simulink model "sampleModel26"  (R2021b)
settings: Solver=VariableStepAuto  StartTime=0.0  StopTime=10.0  RelTol=1e-3
undefined symbols (not defined in the file or in its folder): Newton, Raphson
libraries: simulink x8, slpidlib x4
settings Model: Creator=user  LastModifiedBy=user

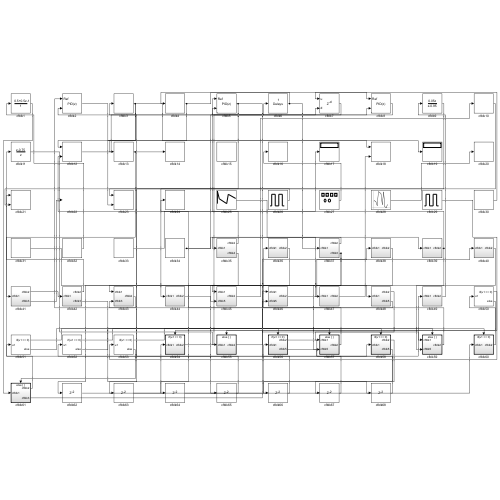
[thumbnail: Simulink's stored preview of the top-level diagram]
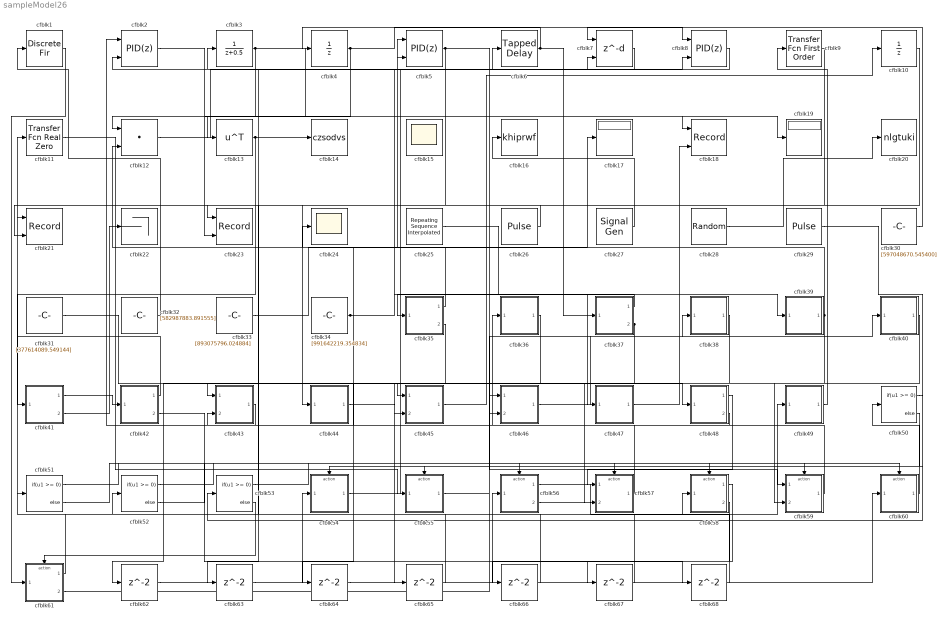
== system sampleModel26 ==
  cfblk1 : DiscreteFir  SampleTime=1
  cfblk10 : UnitDelay  HasFrameUpgradeWarning=on
  cfblk11 : simulink/Discrete/Transfer Fcn Real Zero  ZeroZ=0.75  ICPrevInput=0.0  DoSatur=off
      settings: SourceProductBaseCode=SL
  cfblk12 : DotProduct  InputSameDT=on  OutDataTypeStr=Inherit: Inherit via internal rule
  cfblk13 : Math  Operator=transpose  SaturateOnIntegerOverflow=on
  cfblk14 : ToWorkspace  VariableName=czsodvs  SaveFormat=Timeseries  SampleTime=-1
  cfblk15 : Scope
      settings: Floating=on
  cfblk16 : ToWorkspace  VariableName=khiprwf  SaveFormat=Timeseries  SampleTime=-1
  cfblk17 : Display
  cfblk18 : Record  FileSettingsInternal="{\"entries\":[{\"content\":{\"excelSettings\":{\"content\":{},\"type\":\"Streamout.ExcelSettings\"}},\"type\":\"Streamout.FileSettingStorage\",\"uuid\":\"d4ca884b-6ed6-4891-9e51-d09ac0b6b69e\"}],\"packageUris\":[\"http://schema.mathworks.com/mf0/streamout_blocks/R2020a\"],\"version\":\"1.0\"}"  Layout=[1 1]  SignalsInternal="{\"entries\":[{\"content\":{\"signals\":[{\"content\":{\"blockPath\":[\"sampleModel26/cfblk18\"],\"channel\":[],\"dimensions\":[1,1],\"domain\":\"sampleModel26/cfblk18\",\"lineColor\":\"#a2142f\",\"plots\":[1],\"port\":1,\"sid\":[\"\"],\"signalID\":1005,\"signalName\":\"cfblk3\"},\"type\":\"RecordBlkView.Signal\",\"uuid\":\"a261fcf9-e0b9-45cc-8216-5c8b8619bc2a\"},{\"content\":{\"blockPath\":[\"sampleModel26/cfblk18\"],\"channel\":[],\"dimensions\":[1],\"domain\":\"sampleModel26/cfblk18\",\"lineColor\":\"#139fff\",\"plots\":[1],\"port\":2,\"sid\":[\"\"],\"signalID\":1009,\"signalName\":\"cfblk47\"},\"type\":\"RecordBlkView.Signal\",\"uuid\":\"1b304590-a019-4fec-9271-47d6089c9687\"}]},\"type\":\"RecordBlkView.InputSignals\",\"uuid\":\"9f67ef88-f35c-4418-a645-35f536b90e1d\"}],\"packageUris\":[\"http://schema.mathworks.com/mf0/streamout_blocks/R2020a\"],\"version\":\"1.0\"}"  VisualizationBindings="{\"xyplotplugin\":{\"info\":[{\"series\":[{\"bindingParametersList\":[{\"parameter\":\"X-Axis\",\"signalID\":1005,\"signalName\":\"cfblk3\"},{\"parameter\":\"Y-Axis\",\"signalID\":1009,\"signalName\":\"cfblk47\"}],\"seriesID\":9986}],\"subplotID\":1}]}}"  CompatibilityTag=XY
  cfblk19 : Display
  cfblk2 : slpidlib/PID Controller (2DOF)  Controller=PID  Form=Parallel  TimeDomain=Discrete-time  UseExternalTs=off  SampleTime=1  IntegratorMethod=Forward Euler  FilterMethod=Forward Euler  ControllerParametersSource=internal  P=1  I=1  D=0  UseFilter=on  N=100  b=1  c=1  TunerSelectOption=Transfer Function Based (PID Tuner App)  InitialConditionSource=internal  InitialConditionForIntegrator=0  InitialConditionForFilter=0  DifferentiatorICPrevScaledInput=0  ExternalReset=none  TrackingMode=off  Kt=1  LimitOutput=off  SatLimitsSource=internal  UpperSaturationLimit=inf  LowerSaturationLimit=-inf  LinearizeAsGain=off  AntiWindupMode=none  Kb=1  POutMin=[]  POutMax=[]  IOutMin=[]  IOutMax=[]  DOutMin=[]  DOutMax=[]  NOutMin=[]  NOutMax=[]  bOutMin=[]  bOutMax=[]  cOutMin=[]  cOutMax=[]  SumOutMin=[]  SumOutMax=[]  SaturationOutMin=[]  SaturationOutMax=[]  PParamMin=[]  PParamMax=[]  IParamMin=[]  IParamMax=[]  DParamMin=[]  DParamMax=[]  NParamMin=[]  NParamMax=[]  bParamMin=[]  bParamMax=[]  cParamMin=[]  cParamMax=[]  KbParamMin=[]  KbParamMax=[]  KtParamMin=[]  KtParamMax=[]  KbOutMin=[]  KbOutMax=[]  KtOutMin=[]  KtOutMax=[]  IntegratorOutMin=[]  IntegratorOutMax=[]  FilterOutMin=[]  FilterOutMax=[]  SumI1OutMin=[]  SumI1OutMax=[]  SumI2OutMin=[]  SumI2OutMax=[]  SumI3OutMin=[]  SumI3OutMax=[]  SumI4OutMin=[]  SumI4OutMax=[]  SumDOutMin=[]  SumDOutMax=[]  Sum1OutMin=[]  Sum1OutMax=[]  Sum2OutMin=[]  Sum2OutMax=[]  Sum3OutMin=[]  Sum3OutMax=[]  DifferentiatorOutMin=[]  DifferentiatorOutMax=[]  FilterDiffOutCoefMin=[]  FilterDiffOutCoefMax=[]  ReciprocalOutMin=[]  ReciprocalOutMax=[]  SumDenOutMin=[]  SumDenOutMax=[]  SumNumOutMin=[]  SumNumOutMax=[]  DivideOutMin=[]  DivideOutMax=[]  UdiffTsProdOutMin=[]  UdiffTsProdOutMax=[]  NTsProdOutMin=[]  NTsProdOutMax=[]  UintegralTsProdOutMin=[]  UintegralTsProdOutMax=[]  UngainTsProdOutMin=[]  UngainTsProdOutMax=[]  IntegratorContinuousStateAttributes=''  IntegratorStateMustResolveToSignalObject=off  IntegratorRTWStateStorageClass=Auto  FilterContinuousStateAttributes=''  FilterStateMustResolveToSignalObject=off  FilterRTWStateStorageClass=Auto  ParallelPVariant=InternalParameters  IdealPVariant=Disabled  IVariant=InternalParameters  DVariant=InternalParameters  bVariant=InternalParameters  cVariant=InternalParameters  IntegratorVariant=Discrete  SatVariant=Disabled  AWVariant=Passthrough  PCopyVariant=Disabled  TRVariant=Disabled  FdbkBlocksVariant=Forward  IdealPFdbkVariant=Disabled  SatFdbkVariant=Disabled  DerivativeFilterVariant=ForwardEulerFilter  NVariant=InternalParameters  NCopyVariant=Disabled  FilterICVariant=InternalICsFilter  IntegratorICVariant=InternalICs  ExternalResetVariant=Disabled  TRSumVariant=Passthrough  SumFdbkVariant=Disabled  SumVariant=Sum_PID  TsampFilterVariant=InternalTs  TsampNgainVariant=Passthrough  TsampIntegralVariant=Passthrough  ExternalSaturationOutDataTypeStr=Inherit: Same as second input
      settings: SourceProductBaseCode=SL
  cfblk20 : ToWorkspace  VariableName=nlgtuki  SaveFormat=Timeseries  SampleTime=-1
  cfblk21 : Record  FileSettingsInternal="{\"entries\":[{\"content\":{\"excelSettings\":{\"content\":{},\"type\":\"Streamout.ExcelSettings\"}},\"type\":\"Streamout.FileSettingStorage\",\"uuid\":\"902d94bf-6ad9-4d8d-bb43-3e97950e27a8\"}],\"packageUris\":[\"http://schema.mathworks.com/mf0/streamout_blocks/R2020a\"],\"version\":\"1.0\"}"  Layout=[1 1]  SignalsInternal="{\"entries\":[{\"content\":{\"signals\":[{\"content\":{\"blockPath\":[\"sampleModel26/cfblk21\"],\"channel\":[],\"dimensions\":[1,1],\"domain\":\"sampleModel26/cfblk21\",\"lineColor\":\"#a2142f\",\"plots\":[1],\"port\":1,\"sid\":[\"\"],\"signalID\":1013,\"signalName\":\"cfblk42:1\"},\"type\":\"RecordBlkView.Signal\",\"uuid\":\"12224121-8beb-4598-b1fb-51b9937be4c3\"},{\"content\":{\"blockPath\":[\"sampleModel26/cfblk21\"],\"channel\":[],\"dimensions\":[1],\"domain\":\"sampleModel26/cfblk21\",\"lineColor\":\"#139fff\",\"plots\":[1],\"port\":2,\"sid\":[\"\"],\"signalID\":1017,\"signalName\":\"cfblk10\"},\"type\":\"RecordBlkView.Signal\",\"uuid\":\"13295fa7-14f4-4ec2-bdc1-d2cd68b79197\"}]},\"type\":\"RecordBlkView.InputSignals\",\"uuid\":\"09763a43-9cb4-444a-8828-0097ae43f352\"}],\"packageUris\":[\"http://schema.mathworks.com/mf0/streamout_blocks/R2020a\"],\"version\":\"1.0\"}"  VisualizationBindings="{\"xyplotplugin\":{\"info\":[{\"series\":[{\"bindingParametersList\":[{\"parameter\":\"X-Axis\",\"signalID\":1013,\"signalName\":\"cfblk42:1\"},{\"parameter\":\"Y-Axis\",\"signalID\":1017,\"signalName\":\"cfblk10\"}],\"seriesID\":13624}],\"subplotID\":1}]}}"  CompatibilityTag=XY
  cfblk22 : Terminator
  cfblk23 : Record  FileSettingsInternal="{\"entries\":[{\"content\":{\"excelSettings\":{\"content\":{},\"type\":\"Streamout.ExcelSettings\"}},\"type\":\"Streamout.FileSettingStorage\",\"uuid\":\"a11609d8-2a1b-417e-a440-ff965ac5fa11\"}],\"packageUris\":[\"http://schema.mathworks.com/mf0/streamout_blocks/R2020a\"],\"version\":\"1.0\"}"  Layout=[1 1]  SignalsInternal="{\"entries\":[{\"content\":{\"signals\":[{\"content\":{\"blockPath\":[\"sampleModel26/cfblk23\"],\"channel\":[],\"dimensions\":[1],\"domain\":\"sampleModel26/cfblk23\",\"lineColor\":\"#a2142f\",\"plots\":[1],\"port\":1,\"sid\":[\"\"],\"signalID\":1021,\"signalName\":\"cfblk26\"},\"type\":\"RecordBlkView.Signal\",\"uuid\":\"2700e2c5-e2e7-479b-8112-f551c1b5b9e0\"},{\"content\":{\"blockPath\":[\"sampleModel26/cfblk23\"],\"channel\":[],\"dimensions\":[1,1],\"domain\":\"sampleModel26/cfblk23\",\"lineColor\":\"#139fff\",\"plots\":[1],\"port\":2,\"sid\":[\"\"],\"signalID\":1025,\"signalName\":\"cfblk3\"},\"type\":\"RecordBlkView.Signal\",\"uuid\":\"01e7d8b1-2d56-4034-97cc-cc956fd5e74b\"}]},\"type\":\"RecordBlkView.InputSignals\",\"uuid\":\"823d7022-7059-491d-bee7-1f860ba1237c\"}],\"packageUris\":[\"http://schema.mathworks.com/mf0/streamout_blocks/R2020a\"],\"version\":\"1.0\"}"  VisualizationBindings="{\"xyplotplugin\":{\"info\":[{\"series\":[{\"bindingParametersList\":[{\"parameter\":\"X-Axis\",\"signalID\":1021,\"signalName\":\"cfblk26\"},{\"parameter\":\"Y-Axis\",\"signalID\":1025,\"signalName\":\"cfblk3\"}],\"seriesID\":28488}],\"subplotID\":1}]}}"  CompatibilityTag=XY
  cfblk24 : Scope
  cfblk25 : simulink/Sources/Repeating Sequence Interpolated  OutValues=[-38149698.186429, -442988164.448479, -683927649.777651, -209183975.881470, -429087904.669824]  TimeValues=[0 0.1 0.5 0.6 1].'  LookUpMeth=Interpolation-Use End Values  tsamp=0.01  OutMin=[]  OutMax=[]  OutDataTypeStr=double  OutputDataTypeScalingMode=double  OutDataType=fixdt(0,8)  OutScaling=2^-10
  cfblk26 : DiscretePulseGenerator  PulseType=Time based  Amplitude=[285039313.385840]  Period=[95692373.632031]  PulseWidth=5  PhaseDelay=[2.000000]
  cfblk27 : SignalGenerator  WaveForm=square  Amplitude=[819033828.996605]  Units=rad/sec
  cfblk28 : RandomNumber  Mean=[40847.688215]  Variance=[65157.945720]  Seed=[331896928.000000]  SampleTime=0.1
  cfblk29 : DiscretePulseGenerator  PulseType=Time based  Amplitude=[43137341.195168]  Period=[2476344.846735]  PulseWidth=5  PhaseDelay=[1.000000]
  cfblk3 : DiscreteTransferFcn  SampleTime=1
  cfblk30 : Constant  Value=[597048670.545400]  SampleTime=1
  cfblk31 : Constant  Value=[377614089.549144]  SampleTime=1
  cfblk32 : Constant  Value=[582987883.891555]  SampleTime=1
  cfblk33 : Constant  Value=[893075796.024884]  SampleTime=1
  cfblk34 : Constant  Value=[991642219.354834]  SampleTime=1
  cfblk35 : Subsystem
  cfblk36 : Subsystem
  cfblk37 : Subsystem
  cfblk38 : Subsystem
  cfblk39 : Subsystem
  cfblk4 : UnitDelay  HasFrameUpgradeWarning=on
  cfblk40 : Subsystem
  cfblk41 : Subsystem
  cfblk42 : Subsystem
  cfblk43 : Subsystem
  cfblk44 : Subsystem
  cfblk45 : Subsystem
  cfblk46 : Subsystem
  cfblk47 : Subsystem
  cfblk48 : Subsystem
  cfblk49 : Subsystem
  cfblk5 : slpidlib/PID Controller (2DOF)  Controller=PID  Form=Parallel  TimeDomain=Discrete-time  UseExternalTs=off  SampleTime=1  IntegratorMethod=Forward Euler  FilterMethod=Forward Euler  ControllerParametersSource=internal  P=1  I=1  D=0  UseFilter=on  N=100  b=1  c=1  TunerSelectOption=Transfer Function Based (PID Tuner App)  InitialConditionSource=internal  InitialConditionForIntegrator=0  InitialConditionForFilter=0  DifferentiatorICPrevScaledInput=0  ExternalReset=none  TrackingMode=off  Kt=1  LimitOutput=off  SatLimitsSource=internal  UpperSaturationLimit=inf  LowerSaturationLimit=-inf  LinearizeAsGain=off  AntiWindupMode=none  Kb=1  POutMin=[]  POutMax=[]  IOutMin=[]  IOutMax=[]  DOutMin=[]  DOutMax=[]  NOutMin=[]  NOutMax=[]  bOutMin=[]  bOutMax=[]  cOutMin=[]  cOutMax=[]  SumOutMin=[]  SumOutMax=[]  SaturationOutMin=[]  SaturationOutMax=[]  PParamMin=[]  PParamMax=[]  IParamMin=[]  IParamMax=[]  DParamMin=[]  DParamMax=[]  NParamMin=[]  NParamMax=[]  bParamMin=[]  bParamMax=[]  cParamMin=[]  cParamMax=[]  KbParamMin=[]  KbParamMax=[]  KtParamMin=[]  KtParamMax=[]  KbOutMin=[]  KbOutMax=[]  KtOutMin=[]  KtOutMax=[]  IntegratorOutMin=[]  IntegratorOutMax=[]  FilterOutMin=[]  FilterOutMax=[]  SumI1OutMin=[]  SumI1OutMax=[]  SumI2OutMin=[]  SumI2OutMax=[]  SumI3OutMin=[]  SumI3OutMax=[]  SumI4OutMin=[]  SumI4OutMax=[]  SumDOutMin=[]  SumDOutMax=[]  Sum1OutMin=[]  Sum1OutMax=[]  Sum2OutMin=[]  Sum2OutMax=[]  Sum3OutMin=[]  Sum3OutMax=[]  DifferentiatorOutMin=[]  DifferentiatorOutMax=[]  FilterDiffOutCoefMin=[]  FilterDiffOutCoefMax=[]  ReciprocalOutMin=[]  ReciprocalOutMax=[]  SumDenOutMin=[]  SumDenOutMax=[]  SumNumOutMin=[]  SumNumOutMax=[]  DivideOutMin=[]  DivideOutMax=[]  UdiffTsProdOutMin=[]  UdiffTsProdOutMax=[]  NTsProdOutMin=[]  NTsProdOutMax=[]  UintegralTsProdOutMin=[]  UintegralTsProdOutMax=[]  UngainTsProdOutMin=[]  UngainTsProdOutMax=[]  IntegratorContinuousStateAttributes=''  IntegratorStateMustResolveToSignalObject=off  IntegratorRTWStateStorageClass=Auto  FilterContinuousStateAttributes=''  FilterStateMustResolveToSignalObject=off  FilterRTWStateStorageClass=Auto  ParallelPVariant=InternalParameters  IdealPVariant=Disabled  IVariant=InternalParameters  DVariant=InternalParameters  bVariant=InternalParameters  cVariant=InternalParameters  IntegratorVariant=Discrete  SatVariant=Disabled  AWVariant=Passthrough  PCopyVariant=Disabled  TRVariant=Disabled  FdbkBlocksVariant=Forward  IdealPFdbkVariant=Disabled  SatFdbkVariant=Disabled  DerivativeFilterVariant=ForwardEulerFilter  NVariant=InternalParameters  NCopyVariant=Disabled  FilterICVariant=InternalICsFilter  IntegratorICVariant=InternalICs  ExternalResetVariant=Disabled  TRSumVariant=Passthrough  SumFdbkVariant=Disabled  SumVariant=Sum_PID  TsampFilterVariant=InternalTs  TsampNgainVariant=Passthrough  TsampIntegralVariant=Passthrough  ExternalSaturationOutDataTypeStr=Inherit: Same as second input
      settings: SourceProductBaseCode=SL
  cfblk{50..53} (4 alike) : If  IfExpression=u1 >= 0  SampleTime=1
  cfblk54 : Subsystem  TreatAsAtomicUnit=on
  cfblk55 : Subsystem  TreatAsAtomicUnit=on
  cfblk56 : Subsystem  TreatAsAtomicUnit=on
  cfblk57 : Subsystem  TreatAsAtomicUnit=on
  cfblk58 : Subsystem  TreatAsAtomicUnit=on
  cfblk59 : Subsystem  TreatAsAtomicUnit=on
  cfblk6 : simulink/Discrete/Tapped Delay  vinit=0.0  samptime=-1  NumDelays=1  DelayOrder=Oldest  includeCurrent=off
  cfblk60 : Subsystem  TreatAsAtomicUnit=on
  cfblk61 : Subsystem  TreatAsAtomicUnit=on
  cfblk{62..68} (7 alike) : Delay  SampleTime=1
  cfblk7 : Delay  DelayLengthSource=Input port  SampleTime=1
      settings: InputPortMap=u0,p1
  cfblk8 : slpidlib/PID Controller (2DOF)  Controller=PID  Form=Parallel  TimeDomain=Discrete-time  UseExternalTs=off  SampleTime=1  IntegratorMethod=Forward Euler  FilterMethod=Forward Euler  ControllerParametersSource=internal  P=1  I=1  D=0  UseFilter=on  N=100  b=1  c=1  TunerSelectOption=Transfer Function Based (PID Tuner App)  InitialConditionSource=internal  InitialConditionForIntegrator=0  InitialConditionForFilter=0  DifferentiatorICPrevScaledInput=0  ExternalReset=none  TrackingMode=off  Kt=1  LimitOutput=off  SatLimitsSource=internal  UpperSaturationLimit=inf  LowerSaturationLimit=-inf  LinearizeAsGain=off  AntiWindupMode=none  Kb=1  POutMin=[]  POutMax=[]  IOutMin=[]  IOutMax=[]  DOutMin=[]  DOutMax=[]  NOutMin=[]  NOutMax=[]  bOutMin=[]  bOutMax=[]  cOutMin=[]  cOutMax=[]  SumOutMin=[]  SumOutMax=[]  SaturationOutMin=[]  SaturationOutMax=[]  PParamMin=[]  PParamMax=[]  IParamMin=[]  IParamMax=[]  DParamMin=[]  DParamMax=[]  NParamMin=[]  NParamMax=[]  bParamMin=[]  bParamMax=[]  cParamMin=[]  cParamMax=[]  KbParamMin=[]  KbParamMax=[]  KtParamMin=[]  KtParamMax=[]  KbOutMin=[]  KbOutMax=[]  KtOutMin=[]  KtOutMax=[]  IntegratorOutMin=[]  IntegratorOutMax=[]  FilterOutMin=[]  FilterOutMax=[]  SumI1OutMin=[]  SumI1OutMax=[]  SumI2OutMin=[]  SumI2OutMax=[]  SumI3OutMin=[]  SumI3OutMax=[]  SumI4OutMin=[]  SumI4OutMax=[]  SumDOutMin=[]  SumDOutMax=[]  Sum1OutMin=[]  Sum1OutMax=[]  Sum2OutMin=[]  Sum2OutMax=[]  Sum3OutMin=[]  Sum3OutMax=[]  DifferentiatorOutMin=[]  DifferentiatorOutMax=[]  FilterDiffOutCoefMin=[]  FilterDiffOutCoefMax=[]  ReciprocalOutMin=[]  ReciprocalOutMax=[]  SumDenOutMin=[]  SumDenOutMax=[]  SumNumOutMin=[]  SumNumOutMax=[]  DivideOutMin=[]  DivideOutMax=[]  UdiffTsProdOutMin=[]  UdiffTsProdOutMax=[]  NTsProdOutMin=[]  NTsProdOutMax=[]  UintegralTsProdOutMin=[]  UintegralTsProdOutMax=[]  UngainTsProdOutMin=[]  UngainTsProdOutMax=[]  IntegratorContinuousStateAttributes=''  IntegratorStateMustResolveToSignalObject=off  IntegratorRTWStateStorageClass=Auto  FilterContinuousStateAttributes=''  FilterStateMustResolveToSignalObject=off  FilterRTWStateStorageClass=Auto  ParallelPVariant=InternalParameters  IdealPVariant=Disabled  IVariant=InternalParameters  DVariant=InternalParameters  bVariant=InternalParameters  cVariant=InternalParameters  IntegratorVariant=Discrete  SatVariant=Disabled  AWVariant=Passthrough  PCopyVariant=Disabled  TRVariant=Disabled  FdbkBlocksVariant=Forward  IdealPFdbkVariant=Disabled  SatFdbkVariant=Disabled  DerivativeFilterVariant=ForwardEulerFilter  NVariant=InternalParameters  NCopyVariant=Disabled  FilterICVariant=InternalICsFilter  IntegratorICVariant=InternalICs  ExternalResetVariant=Disabled  TRSumVariant=Passthrough  SumFdbkVariant=Disabled  SumVariant=Sum_PID  TsampFilterVariant=InternalTs  TsampNgainVariant=Passthrough  TsampIntegralVariant=Passthrough  ExternalSaturationOutDataTypeStr=Inherit: Same as second input
      settings: SourceProductBaseCode=SL
  cfblk9 : simulink/Discrete/Transfer Fcn First Order  PoleZ=0.95  ICPrevOutput=0.0  DoSatur=off
  wires:
  cfblk46/1(cfblk2) -> cfblk38/1(cfblk1)
  cfblk57/1(cfblk2) -> cfblk36/1(cfblk1)
  cfblk54/1(cfblk2) -> cfblk6/1
  cfblk45/1(cfblk2) -> cfblk10/1
  cfblk37/1(cfblk2) -> cfblk35/1(cfblk1)
  cfblk28/1 -> cfblk20/1
  cfblk60/1(cfblk2) -> cfblk50/1
  cfblk56/1(cfblk2) -> cfblk49/1(cfblk1)
  cfblk4/1 -> cfblk12/1, cfblk8/1
  cfblk29/1 -> cfblk53/1
  cfblk13/1 -> cfblk14/1, cfblk41/1(cfblk1)
  cfblk34/1 -> cfblk39/1(cfblk1), cfblk8/2
  cfblk37/2(cfblk3) -> cfblk43/1(cfblk1), cfblk57/2(cfblk5)
  cfblk30/1 -> cfblk7/1
  cfblk3/1 -> cfblk18/1, cfblk13/1, cfblk23/2
  cfblk61/1(cfblk2) -> cfblk11/1
  cfblk48/1(cfblk2) -> cfblk57/1(cfblk1)
  cfblk39/1(cfblk2) -> cfblk5/1, cfblk59/2(cfblk5)
  cfblk43/1(cfblk2) -> cfblk2/1
  cfblk12/1 -> cfblk7/2
  cfblk31/1 -> cfblk48/1(cfblk1)
  cfblk55/1(cfblk2) -> cfblk40/1(cfblk1)
  cfblk1/1 -> cfblk61/1(cfblk1)
  cfblk33/1 -> cfblk17/1
  cfblk61/2(cfblk3) -> cfblk46/2(cfblk5)
  cfblk9/1 -> cfblk44/1(cfblk1)
  cfblk56/2(cfblk5) -> cfblk58/1(cfblk1)
  cfblk42/1(cfblk2) -> cfblk21/1
  cfblk59/1(cfblk2) -> cfblk24/1
  cfblk47/1(cfblk2) -> cfblk18/2
  cfblk11/1 -> cfblk55/1(cfblk1)
  cfblk48/2(cfblk5) -> cfblk43/2(cfblk3)
  cfblk5/1 -> cfblk59/1(cfblk1), cfblk63/1
  cfblk32/1 -> cfblk1/1
  cfblk8/1 -> cfblk2/2
  cfblk49/1(cfblk2) -> cfblk9/1
  cfblk40/1(cfblk2) -> cfblk45/1(cfblk1)
  cfblk10/1 -> cfblk21/2
  cfblk41/1(cfblk2) -> cfblk42/1(cfblk1)
  cfblk25/1 -> cfblk47/1(cfblk1)
  cfblk2/1 -> cfblk19/1
  cfblk27/1 -> cfblk16/1
  cfblk7/1 -> cfblk5/2
  cfblk35/1(cfblk2) -> cfblk12/2
  cfblk26/1 -> cfblk23/1
  cfblk6/1 -> cfblk4/1, cfblk37/1(cfblk1)
  cfblk41/2(cfblk3) -> cfblk22/1
  cfblk35/2(cfblk4) -> cfblk45/2(cfblk5)
  cfblk50/1 -> cfblk54/Action
  cfblk50/2 -> cfblk55/Action
  cfblk51/1 -> cfblk56/Action
  cfblk51/2 -> cfblk57/Action
  cfblk52/1 -> cfblk58/Action
  cfblk52/2 -> cfblk59/Action
  cfblk53/1 -> cfblk60/Action
  cfblk53/2 -> cfblk61/Action
  cfblk38/1(cfblk2) -> cfblk62/1
  cfblk62/1 -> cfblk60/1(cfblk1)
  cfblk63/1 -> cfblk54/1(cfblk1)
  cfblk36/1(cfblk2) -> cfblk64/1
  cfblk64/1 -> cfblk56/1(cfblk1)
  cfblk44/1(cfblk2) -> cfblk65/1
  cfblk65/1 -> cfblk51/1
  cfblk58/1(cfblk2) -> cfblk66/1
  cfblk66/1 -> cfblk46/1(cfblk1)
  cfblk58/2(cfblk5) -> cfblk67/1
  cfblk67/1 -> cfblk52/1
  cfblk42/2(cfblk3) -> cfblk68/1
  cfblk68/1 -> cfblk3/1

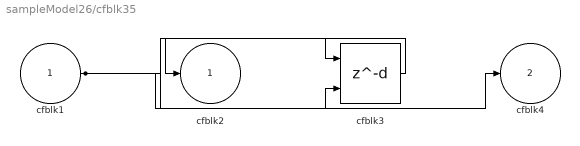
== system sampleModel26/cfblk35 ==
  cfblk1 : Inport
  cfblk3 : Delay  DelayLengthSource=Input port  SampleTime=1
      settings: InputPortMap=u0,p1
  cfblk2 : Outport
  cfblk4 : Outport  Port=2
  wires:
  cfblk3/1 -> cfblk2/1
  cfblk1/1 -> cfblk4/1, cfblk3/1, cfblk3/2

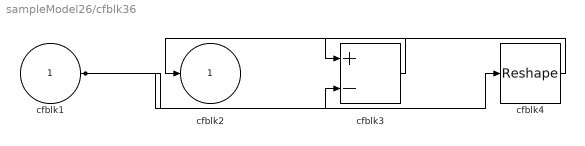
== system sampleModel26/cfblk36 ==
  cfblk1 : Inport
  cfblk3 : Sum  Inputs=+-
  cfblk4 : Reshape
  cfblk2 : Outport
  wires:
  cfblk3/1 -> cfblk2/1
  cfblk1/1 -> cfblk4/1, cfblk3/2
  cfblk4/1 -> cfblk3/1

== system sampleModel26/cfblk37 ==
  cfblk1 : Inport
  cfblk2 : Outport
  cfblk3 : Outport  Port=2
  wires:
  cfblk1/1 -> cfblk3/1, cfblk2/1

== system sampleModel26/cfblk38 ==
  cfblk1 : Inport
  cfblk3 : slpidlib/PID Controller  Controller=PID  Form=Parallel  TimeDomain=Discrete-time  UseExternalTs=off  SampleTime=1  IntegratorMethod=Forward Euler  FilterMethod=Forward Euler  ControllerParametersSource=internal  P=1  I=1  D=0  UseFilter=on  N=100  TunerSelectOption=Transfer Function Based (PID Tuner App)  InitialConditionSource=internal  InitialConditionForIntegrator=0  InitialConditionForFilter=0  DifferentiatorICPrevScaledInput=0  ExternalReset=none  TrackingMode=off  Kt=1  LimitOutput=off  SatLimitsSource=internal  UpperSaturationLimit=inf  LowerSaturationLimit=-inf  LinearizeAsGain=off  AntiWindupMode=none  Kb=1  POutMin=[]  POutMax=[]  IOutMin=[]  IOutMax=[]  DOutMin=[]  DOutMax=[]  NOutMin=[]  NOutMax=[]  SumOutMin=[]  SumOutMax=[]  SaturationOutMin=[]  SaturationOutMax=[]  PParamMin=[]  PParamMax=[]  IParamMin=[]  IParamMax=[]  DParamMin=[]  DParamMax=[]  NParamMin=[]  NParamMax=[]  KbParamMin=[]  KbParamMax=[]  KtParamMin=[]  KtParamMax=[]  KbOutMin=[]  KbOutMax=[]  KtOutMin=[]  KtOutMax=[]  IntegratorOutMin=[]  IntegratorOutMax=[]  FilterOutMin=[]  FilterOutMax=[]  SumI1OutMin=[]  SumI1OutMax=[]  SumI2OutMin=[]  SumI2OutMax=[]  SumI3OutMin=[]  SumI3OutMax=[]  SumI4OutMin=[]  SumI4OutMax=[]  SumDOutMin=[]  SumDOutMax=[]  DifferentiatorOutMin=[]  DifferentiatorOutMax=[]  FilterDiffOutCoefMin=[]  FilterDiffOutCoefMax=[]  ReciprocalOutMin=[]  ReciprocalOutMax=[]  SumDenOutMin=[]  SumDenOutMax=[]  SumNumOutMin=[]  SumNumOutMax=[]  DivideOutMin=[]  DivideOutMax=[]  UdiffTsProdOutMin=[]  UdiffTsProdOutMax=[]  NTsProdOutMin=[]  NTsProdOutMax=[]  UintegralTsProdOutMin=[]  UintegralTsProdOutMax=[]  UngainTsProdOutMin=[]  UngainTsProdOutMax=[]  IntegratorContinuousStateAttributes=''  IntegratorStateMustResolveToSignalObject=off  IntegratorRTWStateStorageClass=Auto  FilterContinuousStateAttributes=''  FilterStateMustResolveToSignalObject=off  FilterRTWStateStorageClass=Auto  ParallelPVariant=InternalParameters  IdealPVariant=Disabled  IVariant=InternalParameters  DVariant=InternalParameters  IntegratorVariant=Discrete  SatVariant=Disabled  AWVariant=Passthrough  PCopyVariant=Disabled  TRVariant=Disabled  FdbkBlocksVariant=Forward  IdealPFdbkVariant=Disabled  SatFdbkVariant=Disabled  DerivativeFilterVariant=ForwardEulerFilter  NVariant=InternalParameters  NCopyVariant=Disabled  FilterICVariant=InternalICsFilter  IntegratorICVariant=InternalICs  ExternalResetVariant=Disabled  TRSumVariant=Passthrough  SumFdbkVariant=Disabled  SumVariant=Sum_PID  TsampFilterVariant=InternalTs  TsampNgainVariant=Passthrough  TsampIntegralVariant=Passthrough  ExternalSaturationOutDataTypeStr=Inherit: Same as second input
  cfblk2 : Outport
  wires:
  cfblk1/1 -> cfblk3/1
  cfblk3/1 -> cfblk2/1

== system sampleModel26/cfblk39 ==
  cfblk1 : Inport
  cfblk3 : ComplexToMagnitudeAngle
  cfblk2 : Outport
  wires:
  cfblk1/1 -> cfblk3/1
  cfblk3/1 -> cfblk2/1

== system sampleModel26/cfblk40 ==
  cfblk1 : Inport
  cfblk3 : Sqrt  Operator=rSqrt  AlgorithmType=Newton-Raphson  SaturateOnIntegerOverflow=on
  cfblk4 : Constant  Value=[-667124386.739958]  SampleTime=1
  cfblk2 : Outport
  wires:
  cfblk1/1 -> cfblk3/1
  cfblk4/1 -> cfblk2/1

== system sampleModel26/cfblk41 ==
  cfblk1 : Inport
  cfblk2 : Outport
  cfblk3 : Outport  Port=2
  wires:
  cfblk1/1 -> cfblk2/1, cfblk3/1

== system sampleModel26/cfblk42 ==
  cfblk1 : Inport
  cfblk2 : Outport
  cfblk3 : Outport  Port=2
  wires:
  cfblk1/1 -> cfblk2/1, cfblk3/1

== system sampleModel26/cfblk43 ==
  cfblk1 : Inport
  cfblk3 : Inport  Port=2
  cfblk2 : Outport
  wires:
  cfblk1/1 -> cfblk2/1

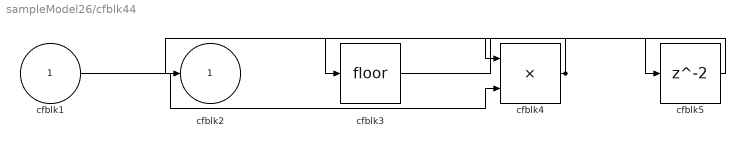
== system sampleModel26/cfblk44 ==
  cfblk1 : Inport
  cfblk3 : Rounding
  cfblk4 : Product
  cfblk5 : Delay  SampleTime=1
  cfblk2 : Outport
  wires:
  cfblk1/1 -> cfblk4/2
  cfblk4/1 -> cfblk2/1, cfblk3/1
  cfblk3/1 -> cfblk5/1
  cfblk5/1 -> cfblk4/1

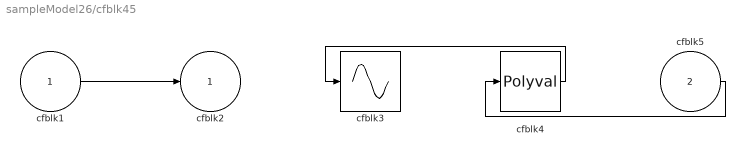
== system sampleModel26/cfblk45 ==
  cfblk1 : Inport
  cfblk5 : Inport  Port=2
  cfblk3 : Sin  TimeSource=Use external signal  SampleTime=0
  cfblk4 : Polyval  Coefs=[ +2.081618890e-019, -1.441693666e-014, +4.719686976e-010, -8.536869453e-006, +1.621573104e-001, -8.087801117e+001 ]
  cfblk2 : Outport
  wires:
  cfblk4/1 -> cfblk3/1
  cfblk1/1 -> cfblk2/1
  cfblk5/1 -> cfblk4/1

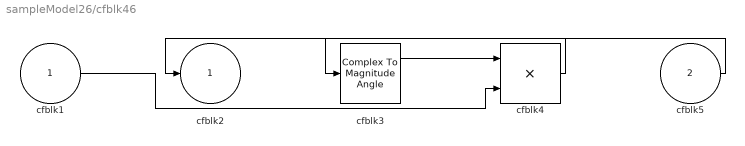
== system sampleModel26/cfblk46 ==
  cfblk1 : Inport
  cfblk5 : Inport  Port=2
  cfblk3 : ComplexToMagnitudeAngle
  cfblk4 : Product  Inputs=**
  cfblk2 : Outport
  wires:
  cfblk3/1 -> cfblk4/1
  cfblk4/1 -> cfblk2/1
  cfblk1/1 -> cfblk4/2
  cfblk5/1 -> cfblk3/1

== system sampleModel26/cfblk47 ==
  cfblk1 : Inport
  cfblk3 : Sum  Inputs=+-
  cfblk2 : Outport
  wires:
  cfblk1/1 -> cfblk3/1, cfblk3/2
  cfblk3/1 -> cfblk2/1

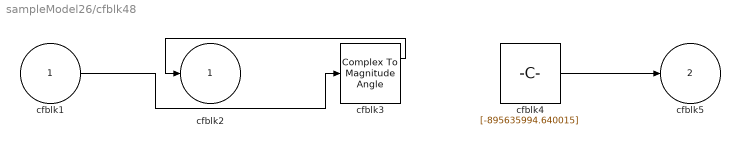
== system sampleModel26/cfblk48 ==
  cfblk1 : Inport
  cfblk3 : ComplexToMagnitudeAngle
  cfblk4 : Constant  Value=[-895635994.640015]  SampleTime=1
  cfblk2 : Outport
  cfblk5 : Outport  Port=2
  wires:
  cfblk3/1 -> cfblk2/1
  cfblk1/1 -> cfblk3/1
  cfblk4/1 -> cfblk5/1

== system sampleModel26/cfblk49 ==
  cfblk1 : Inport
  cfblk3 : DiscreteZeroPole  Poles=[0 0.5]  Gain=1
  cfblk2 : Outport
  wires:
  cfblk3/1 -> cfblk2/1
  cfblk1/1 -> cfblk3/1

== system sampleModel26/cfblk54 ==
  cfblk1 : Inport
  Action Port : ActionPort  ActionPortLabel=if(u1 >= 0)
  cfblk3 : simulink/Discrete/Difference  ICPrevInput=0.0  OutMin=[]  OutMax=[]  OutDataTypeStr=Inherit: Inherit via back propagation  OutDataType=fixdt(1, 16)  OutScaling=2^-10  DoSatur=off
  cfblk2 : Outport
  wires:
  cfblk1/1 -> cfblk3/1
  cfblk3/1 -> cfblk2/1

== system sampleModel26/cfblk55 ==
  cfblk1 : Inport
  Action Port : ActionPort  ActionPortLabel=else
  cfblk3 : Trigonometry
  cfblk2 : Outport
  wires:
  cfblk3/1 -> cfblk2/1
  cfblk1/1 -> cfblk3/1

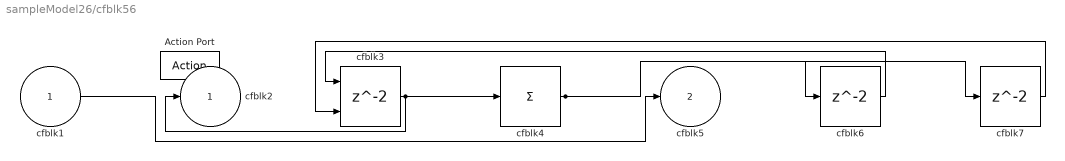
== system sampleModel26/cfblk56 ==
  cfblk1 : Inport
  Action Port : ActionPort  ActionPortLabel=if(u1 >= 0)
  cfblk3 : Delay  ShowEnablePort=on
      settings: InputPortMap=u0,e6
  cfblk4 : Sum  Inputs=+
  cfblk6 : Delay
  cfblk7 : Delay
  cfblk2 : Outport
  cfblk5 : Outport  Port=2
  wires:
  cfblk3/1 -> cfblk2/1, cfblk4/1
  cfblk4/1 -> cfblk6/1, cfblk7/1
  cfblk1/1 -> cfblk5/1
  cfblk6/1 -> cfblk3/1
  cfblk7/1 -> cfblk3/2

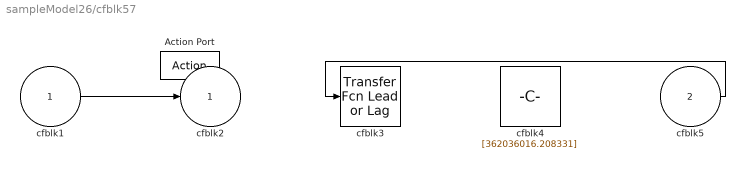
== system sampleModel26/cfblk57 ==
  cfblk1 : Inport
  cfblk5 : Inport  Port=2
  Action Port : ActionPort  ActionPortLabel=else
  cfblk3 : simulink/Discrete/Transfer Fcn Lead or Lag  PoleZ=0.95  ZeroZ=0.75  ICPrevOutput=0.0  ICPrevInput=0.0  DoSatur=off
      settings: SourceProductBaseCode=SL
  cfblk4 : Constant  Value=[362036016.208331]  SampleTime=1
  cfblk2 : Outport
  wires:
  cfblk1/1 -> cfblk2/1
  cfblk5/1 -> cfblk3/1

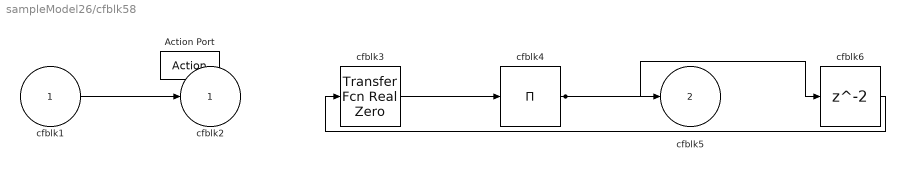
== system sampleModel26/cfblk58 ==
  cfblk1 : Inport
  Action Port : ActionPort  ActionPortLabel=if(u1 >= 0)
  cfblk3 : simulink/Discrete/Transfer Fcn Real Zero  ZeroZ=0.75  ICPrevInput=0.0  DoSatur=off
      settings: SourceProductBaseCode=SL
  cfblk4 : Product  Inputs=*
  cfblk6 : Delay
  cfblk2 : Outport
  cfblk5 : Outport  Port=2
  wires:
  cfblk4/1 -> cfblk5/1, cfblk6/1
  cfblk1/1 -> cfblk2/1
  cfblk3/1 -> cfblk4/1
  cfblk6/1 -> cfblk3/1

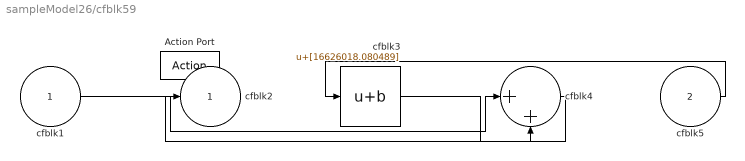
== system sampleModel26/cfblk59 ==
  cfblk1 : Inport
  cfblk5 : Inport  Port=2
  Action Port : ActionPort  ActionPortLabel=else
  cfblk3 : Bias  Bias=[16626018.080489]
  cfblk4 : Sum  Inputs=|++
  cfblk2 : Outport
  wires:
  cfblk1/1 -> cfblk4/1
  cfblk4/1 -> cfblk2/1
  cfblk5/1 -> cfblk3/1
  cfblk3/1 -> cfblk4/2

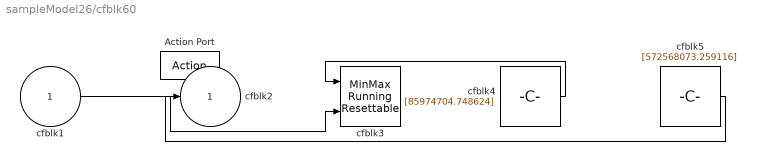
== system sampleModel26/cfblk60 ==
  cfblk1 : Inport
  Action Port : ActionPort  ActionPortLabel=if(u1 >= 0)
  cfblk3 : simulink/Math Operations/MinMax Running Resettable  Function=min  vinit=0.0
  cfblk4 : Constant  Value=[85974704.748624]  SampleTime=1
  cfblk5 : Constant  Value=[572568073.259116]  SampleTime=1
  cfblk2 : Outport
  wires:
  cfblk4/1 -> cfblk3/1
  cfblk1/1 -> cfblk3/2
  cfblk5/1 -> cfblk2/1

== system sampleModel26/cfblk61 ==
  cfblk1 : Inport
  Action Port : ActionPort  ActionPortLabel=else
  cfblk2 : Outport
  cfblk3 : Outport  Port=2
  wires:
  cfblk1/1 -> cfblk3/1, cfblk2/1
